simulink model "model"  (R2016b)
settings: Solver=VariableStepAuto  StartTime=0.0  StopTime=5  RelTol=1e-3
undefined symbols (not defined in the file): K, Kv, T1, T2, w1, w2, w3
settings Model: Creator=senserlex  LastModifiedBy=senserlex
settings DataIOCC: LimitDataPoints=on  SaveOutput=off  SaveTime=off
settings OptimizationCC: BlockReduction=off  BooleanDataType=off  LifeSpan=inf
settings DebuggingCC: SaveWithParameterizedLinksMsg=none  UnderspecifiedInitializationDetection=Classic  MergeDetectMultiDrivingBlocksExec=none  SignalResolutionControl=TryResolveAllWithWarning  AllowSymbolicDim=off  SFUnexpectedBacktrackingDiag=warning  SFNoUnconditionalDefaultTransitionDiag=warning  SFExecutionAtInitializationDiag=none
settings HardwareCC: TargetUnknown=on
settings GRTTargetCC: TargetLangStandard=C89/C90 (ANSI)  GeneratePreprocessorConditionals=Disable all

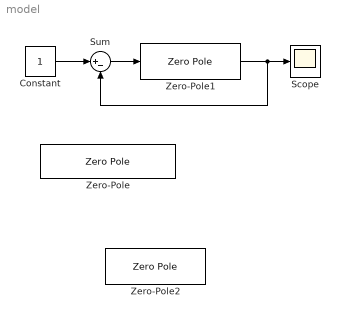
== system model ==
  Constant : Constant
  Scope : Scope
  Sum : Sum  Inputs=|+-
  Zero-Pole : ZeroPole  Zeros=[-w2 -1/T1 -1/T2]  Poles=[-w1 -w3 -w3]  Gain=[Kv/K]
  Zero-Pole1 : ZeroPole  Zeros=[ ]  Poles=[-1/T1 -1/T2 0]  Gain=[K/(T1*T2)]
  Zero-Pole2 : ZeroPole  Zeros=[-w2]  Poles=[0 -w1 -w3 -w3]  Gain=[Kv]
  wires:
  Constant/1 -> Sum/1
  Sum/1 -> Zero-Pole1/1
  Zero-Pole1/1 -> Sum/2, Scope/1
